simulink model "pendulo"  (R2019b)
settings: Solver=ode45  StartTime=0  StopTime=inf  MaxStep=0.02  RelTol=1e-3  AbsTol=1e-6
libraries: neural x76, simulink x2
(part 2 of 4)

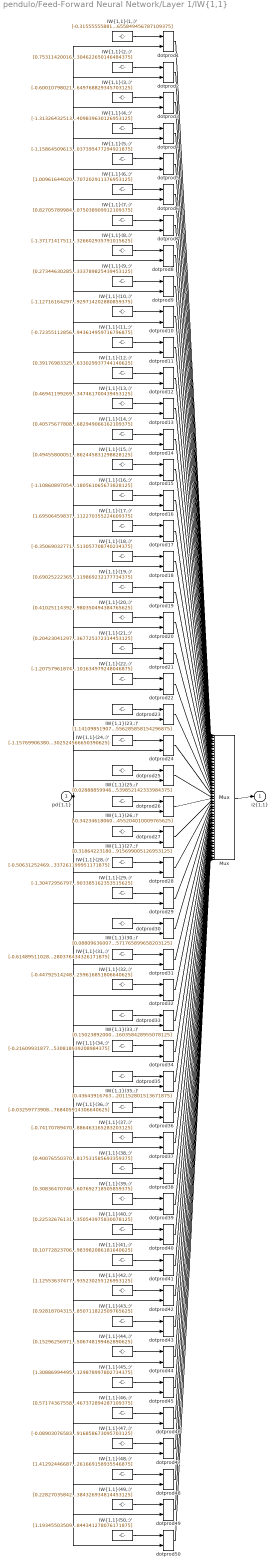
== system pendulo/Feed-Forward Neural Network/Layer 1/IW{1,1} ==
  "pd{1,1}" : Inport  PortDimensions=9
      mask Display: e = 0.06;c1 = [120 230 180]/255;c2 = ([120 230 180]+0)/(256+128);c3 = ([120 230 180]+128)/(256+128);patch([0 1 1 0],[0 0 1 1],c1);patch([0 1 1 1-e 1-e 0+e],[0 0 1 1-e 0+e 0+e],c2);patch([0 0 1 1-e 0+e 0+e],[0 1 1 1-e 1-e 0+e],c3);plot([0 1 1 0 0],[0 0 1 1 0]);
  "IW{1,1}(1,:)'" : Constant  Value=[-0.31555555881384067529182857470004819333553314208984375;0.42878021754571926660304370670928619801998138427734375;-0.0107473012178736886113039616930109332315623760223388671875;-1.3786333332536795381884076050482690334320068359375;0.2466842726358048076829021511002792976796627044677734375;-0.443770337362677957937506789676262997090816497802734375;0.6142590886963574803303345106542110443115234375;0.79347793333041438668118416899233125150203704833984375;0.484092147104690118109004970392561517655849456787109375]
      mask Display: e = 0.06;c1 = [120 150 230]/255;c2 = ([120 150 230]+0)/383;c3 = ([120 150 230]+128)/383;patch([0 1 1 0],[0 0 1 1],c1);patch([0 1 1 1-e 1-e 0+e],[0 0 1 1-e 0+e 0+e],c2);patch([0 0 1 1-e 0+e 0+e],[0 1 1 1-e 1-e 0+e],c3);plot([0 1 1 0 0],[0 0 1 1 0]);disp('Weights');
  "IW{1,1}(10,:)'" : Constant  Value=[-1.127161642979468414438315448933281004428863525390625;-0.01531473256999515801524136549005561391822993755340576171875;0.66738346115575308825640377108356915414333343505859375;0.9754438276149068887121984516852535307407379150390625;-0.9679253878951674661124116028076969087123870849609375;0.733607171987361805776117762434296309947967529296875;0.57226531948503878144407508443691767752170562744140625;-0.931214454864173202253141425899229943752288818359375;0.39431807532208207334178950986824929714202880859375]
      mask Display: e = 0.06;c1 = [120 150 230]/255;c2 = ([120 150 230]+0)/383;c3 = ([120 150 230]+128)/383;patch([0 1 1 0],[0 0 1 1],c1);patch([0 1 1 1-e 1-e 0+e],[0 0 1 1-e 0+e 0+e],c2);patch([0 0 1 1-e 0+e 0+e],[0 1 1 1-e 1-e 0+e],c3);plot([0 1 1 0 0],[0 0 1 1 0]);disp('Weights');
  "IW{1,1}(11,:)'" : Constant  Value=[-0.7235511285626261557268890101113356649875640869140625;-1.1538311728051569016173516502021811902523040771484375;0.83219382713551415253760978885111398994922637939453125;0.8528391957357628339053690069704316556453704833984375;-1.225194887015537137386900212732143700122833251953125;-0.113464709832653609655750415186048485338687896728515625;-0.65765666929837907073164160465239547193050384521484375;-0.6645356436380531750529598866705782711505889892578125;-0.144071189137995492313137901874142698943614959716796875]
      mask Display: e = 0.06;c1 = [120 150 230]/255;c2 = ([120 150 230]+0)/383;c3 = ([120 150 230]+128)/383;patch([0 1 1 0],[0 0 1 1],c1);patch([0 1 1 1-e 1-e 0+e],[0 0 1 1-e 0+e 0+e],c2);patch([0 0 1 1-e 0+e 0+e],[0 1 1 1-e 1-e 0+e],c3);plot([0 1 1 0 0],[0 0 1 1 0]);disp('Weights');
  "IW{1,1}(12,:)'" : Constant  Value=[0.39176983325826231219224382584798149764537811279296875;-0.30969059820905975310978419656748883426189422607421875;-0.157098741820563658766474190997541882097721099853515625;-0.734606532386577359972079648287035524845123291015625;0.2214909422180497688970035596867091953754425048828125;1.28271197347724363879706288571469485759735107421875;0.53025793193026615757190711519797332584857940673828125;0.8886386670511843277608932112343609333038330078125;0.20817546322240121359214981566765345633029937744140625]
      mask Display: e = 0.06;c1 = [120 150 230]/255;c2 = ([120 150 230]+0)/383;c3 = ([120 150 230]+128)/383;patch([0 1 1 0],[0 0 1 1],c1);patch([0 1 1 1-e 1-e 0+e],[0 0 1 1-e 0+e 0+e],c2);patch([0 0 1 1-e 0+e 0+e],[0 1 1 1-e 1-e 0+e],c3);plot([0 1 1 0 0],[0 0 1 1 0]);disp('Weights');
  "IW{1,1}(13,:)'" : Constant  Value=[0.4694119926947788457027854747138917446136474609375;0.84304552135569787996161039700382389128208160400390625;-0.56604187158333540974552988700452260673046112060546875;0.12057132118322488878447984461672604084014892578125;1.928569665412307898577637388370931148529052734375;-0.676114380799501812902008168748579919338226318359375;0.239362492717263009023298536703805439174175262451171875;0.10001219768902032403179447328511741943657398223876953125;-1.3863310520411193937917460061726160347461700439453125]
      mask Display: e = 0.06;c1 = [120 150 230]/255;c2 = ([120 150 230]+0)/383;c3 = ([120 150 230]+128)/383;patch([0 1 1 0],[0 0 1 1],c1);patch([0 1 1 1-e 1-e 0+e],[0 0 1 1-e 0+e 0+e],c2);patch([0 0 1 1-e 0+e 0+e],[0 1 1 1-e 1-e 0+e],c3);plot([0 1 1 0 0],[0 0 1 1 0]);disp('Weights');
  "IW{1,1}(14,:)'" : Constant  Value=[0.405756778086816483064325211671530269086360931396484375;1.4762826494711440705742688805912621319293975830078125;-0.6160052014403716302837210605503059923648834228515625;0.370993442519975957782918385419179685413837432861328125;0.5321273006076394640473381514311768114566802978515625;-0.63250490898227551550547786973766051232814788818359375;0.1763096386724627706588108821961213834583759307861328125;-0.002711608591991353407746334625016970676369965076446533203125;-0.5335206946245099057790639562881551682949066162109375]
      mask Display: e = 0.06;c1 = [120 150 230]/255;c2 = ([120 150 230]+0)/383;c3 = ([120 150 230]+128)/383;patch([0 1 1 0],[0 0 1 1],c1);patch([0 1 1 1-e 1-e 0+e],[0 0 1 1-e 0+e 0+e],c2);patch([0 0 1 1-e 0+e 0+e],[0 1 1 1-e 1-e 0+e],c3);plot([0 1 1 0 0],[0 0 1 1 0]);disp('Weights');
  "IW{1,1}(15,:)'" : Constant  Value=[0.4945580005144349922119317852775566279888153076171875;-0.30371329537800229037003418852691538631916046142578125;-0.12657247648842939735658319477806799113750457763671875;-1.254771661749214839431942891678772866725921630859375;1.2513953241071182898025426766253076493740081787109375;-0.2429382434092005327297414396525709889829158782958984375;-0.9021522058858228998445838442421518266201019287109375;-0.71761308572964221941248297298443503677845001220703125;0.59448766002498942828680128513951785862445831298828125]
      mask Display: e = 0.06;c1 = [120 150 230]/255;c2 = ([120 150 230]+0)/383;c3 = ([120 150 230]+128)/383;patch([0 1 1 0],[0 0 1 1],c1);patch([0 1 1 1-e 1-e 0+e],[0 0 1 1-e 0+e 0+e],c2);patch([0 0 1 1-e 0+e 0+e],[0 1 1 1-e 1-e 0+e],c3);plot([0 1 1 0 0],[0 0 1 1 0]);disp('Weights');
  "IW{1,1}(16,:)'" : Constant  Value=[-1.1086089705421182660671775010996498167514801025390625;0.13153072035216284429992583682178519666194915771484375;0.188915927396714977692937509345938451588153839111328125;-0.8110236400015413682496046021697111427783966064453125;-0.383791213781895346190964346533291973173618316650390625;0.0019837883702850493683467192340685869567096233367919921875;0.68049020551012129320866961279534734785556793212890625;1.2210924520571777573962890528491698205471038818359375;0.9901086444778670614397242388804443180561065673828125]
      mask Display: e = 0.06;c1 = [120 150 230]/255;c2 = ([120 150 230]+0)/383;c3 = ([120 150 230]+128)/383;patch([0 1 1 0],[0 0 1 1],c1);patch([0 1 1 1-e 1-e 0+e],[0 0 1 1-e 0+e 0+e],c2);patch([0 0 1 1-e 0+e 0+e],[0 1 1 1-e 1-e 0+e],c3);plot([0 1 1 0 0],[0 0 1 1 0]);disp('Weights');
  "IW{1,1}(17,:)'" : Constant  Value=[1.695064598379282916340571318869479000568389892578125;0.37882205685793424176921462276368401944637298583984375;0.400870413159026328653311566085903905332088470458984375;-2.0781413995163919850028833025135099887847900390625;1.73490465554027384342816731077618896961212158203125;-1.444554989619908358378097545937635004520416259765625;1.521775698019746325684309340431354939937591552734375;-1.146726490581089219489285824238322675228118896484375;-0.1395995298359869740689731543170637451112270355224609375]
      mask Display: e = 0.06;c1 = [120 150 230]/255;c2 = ([120 150 230]+0)/383;c3 = ([120 150 230]+128)/383;patch([0 1 1 0],[0 0 1 1],c1);patch([0 1 1 1-e 1-e 0+e],[0 0 1 1-e 0+e 0+e],c2);patch([0 0 1 1-e 0+e 0+e],[0 1 1 1-e 1-e 0+e],c3);plot([0 1 1 0 0],[0 0 1 1 0]);disp('Weights');
  "IW{1,1}(18,:)'" : Constant  Value=[-0.350690327718819194746657785799470730125904083251953125;-0.7298307839542406139088370764511637389659881591796875;0.080331001842342708574307152957771904766559600830078125;-0.2264533897417844443555878797269542701542377471923828125;1.2103384853547785038330175666487775743007659912109375;-0.01487761549236282614117055089764107833616435527801513671875;-1.804827730506363803186786753940396010875701904296875;-0.6133682207425008581225256421021185815334320068359375;-1.1075147321910046027682028579874895513057708740234375]
      mask Display: e = 0.06;c1 = [120 150 230]/255;c2 = ([120 150 230]+0)/383;c3 = ([120 150 230]+128)/383;patch([0 1 1 0],[0 0 1 1],c1);patch([0 1 1 1-e 1-e 0+e],[0 0 1 1-e 0+e 0+e],c2);patch([0 0 1 1-e 0+e 0+e],[0 1 1 1-e 1-e 0+e],c3);plot([0 1 1 0 0],[0 0 1 1 0]);disp('Weights');
  "IW{1,1}(19,:)'" : Constant  Value=[0.69025222365466232243846889105043374001979827880859375;0.72407871395070666498128275634371675550937652587890625;-0.9153915604214015733219866888248361647129058837890625;-0.82307459957225870272878864852827973663806915283203125;-0.2295515018585499722458820315296179614961147308349609375;-0.020777463007284745211133980546946986578404903411865234375;-1.7020463564167707115615257862373255193233489990234375;-0.64572237449823177701802023875643499195575714111328125;-0.019957265337930261972498868772163405083119869232177734375]
      mask Display: e = 0.06;c1 = [120 150 230]/255;c2 = ([120 150 230]+0)/383;c3 = ([120 150 230]+128)/383;patch([0 1 1 0],[0 0 1 1],c1);patch([0 1 1 1-e 1-e 0+e],[0 0 1 1-e 0+e 0+e],c2);patch([0 0 1 1-e 0+e 0+e],[0 1 1 1-e 1-e 0+e],c3);plot([0 1 1 0 0],[0 0 1 1 0]);disp('Weights');
  "IW{1,1}(2,:)'" : Constant  Value=[0.75311420016744168304256845658528618514537811279296875;0.79978875953749961613681307426304556429386138916015625;0.96009154060472201575038297960418276488780975341796875;-0.300561830203671165318013436262845061719417572021484375;0.40602009911398384556235896525322459638118743896484375;1.1108934598249404768210979455034248530864715576171875;0.11083407343756877805329708053250215016305446624755859375;1.558741230264542476646738577983342111110687255859375;-0.8332669372419319042677443576394580304622650146484375]
      mask Display: e = 0.06;c1 = [120 150 230]/255;c2 = ([120 150 230]+0)/383;c3 = ([120 150 230]+128)/383;patch([0 1 1 0],[0 0 1 1],c1);patch([0 1 1 1-e 1-e 0+e],[0 0 1 1-e 0+e 0+e],c2);patch([0 0 1 1-e 0+e 0+e],[0 1 1 1-e 1-e 0+e],c3);plot([0 1 1 0 0],[0 0 1 1 0]);disp('Weights');
  "IW{1,1}(20,:)'" : Constant  Value=[0.41025114392726724776849778208998031914234161376953125;-0.94407653012080505749992198616382665932178497314453125;-0.47173289343233426595958235338912345468997955322265625;1.3654696510674215748082360732951201498508453369140625;-0.104760883286913741851975601093727163970470428466796875;1.648557662635401044326499686576426029205322265625;-2.283586288340160752596830207039602100849151611328125;0.78062908761209881536302646054537035524845123291015625;-0.46100003044116155681564350743428803980350494384765625]
      mask Display: e = 0.06;c1 = [120 150 230]/255;c2 = ([120 150 230]+0)/383;c3 = ([120 150 230]+128)/383;patch([0 1 1 0],[0 0 1 1],c1);patch([0 1 1 1-e 1-e 0+e],[0 0 1 1-e 0+e 0+e],c2);patch([0 0 1 1-e 0+e 0+e],[0 1 1 1-e 1-e 0+e],c3);plot([0 1 1 0 0],[0 0 1 1 0]);disp('Weights');
  "IW{1,1}(21,:)'" : Constant  Value=[0.204230412979091335845538424109690822660923004150390625;0.488765287185259966751260662931599654257297515869140625;-0.95418031643023704102546389549388550221920013427734375;0.82964132894869724310638048336841166019439697265625;0.36653691493746032303846504873945377767086029052734375;1.70232992659664006396269542165100574493408203125;-0.37295451432827542159742506555630825459957122802734375;0.383819067928140522649727017778786830604076385498046875;1.0682066467828168487841367095825262367725372314453125]
      mask Display: e = 0.06;c1 = [120 150 230]/255;c2 = ([120 150 230]+0)/383;c3 = ([120 150 230]+128)/383;patch([0 1 1 0],[0 0 1 1],c1);patch([0 1 1 1-e 1-e 0+e],[0 0 1 1-e 0+e 0+e],c2);patch([0 0 1 1-e 0+e 0+e],[0 1 1 1-e 1-e 0+e],c3);plot([0 1 1 0 0],[0 0 1 1 0]);disp('Weights');
  "IW{1,1}(22,:)'" : Constant  Value=[-1.2075796187402361159257679901202209293842315673828125;-1.4344767144320462737283605747506953775882720947265625;-0.385734577372322584576380677390261553227901458740234375;-0.368066024648789624773570494653540663421154022216796875;1.25235491089850103918479362619109451770782470703125;1.395404085665501003887811748427338898181915283203125;0.7191071159702386861312106702825985848903656005859375;0.37835364418729000579588728214730508625507354736328125;-0.55481502754330758175882465366157703101634979248046875]
      mask Display: e = 0.06;c1 = [120 150 230]/255;c2 = ([120 150 230]+0)/383;c3 = ([120 150 230]+128)/383;patch([0 1 1 0],[0 0 1 1],c1);patch([0 1 1 1-e 1-e 0+e],[0 0 1 1-e 0+e 0+e],c2);patch([0 0 1 1-e 0+e 0+e],[0 1 1 1-e 1-e 0+e],c3);plot([0 1 1 0 0],[0 0 1 1 0]);disp('Weights');
  "IW{1,1}(23,:)'" : Constant  Value=[1.141098519073533879009119118563830852508544921875;-0.7222178307753706061333787147304974496364593505859375;-1.0486600899619560323117184452712535858154296875;-0.9834664350422215317593099825899116694927215576171875;0.27914584816355214602623391328961588442325592041015625;-3.002461764557355916593905931222252547740936279296875;0.79946594802184234307418364551267586648464202880859375;-0.291064075115631981649499948616721667349338531494140625;0.266729788638156495306219539997982792556285858154296875]
      mask Display: e = 0.06;c1 = [120 150 230]/255;c2 = ([120 150 230]+0)/383;c3 = ([120 150 230]+128)/383;patch([0 1 1 0],[0 0 1 1],c1);patch([0 1 1 1-e 1-e 0+e],[0 0 1 1-e 0+e 0+e],c2);patch([0 0 1 1-e 0+e 0+e],[0 1 1 1-e 1-e 0+e],c3);plot([0 1 1 0 0],[0 0 1 1 0]);disp('Weights');
  "IW{1,1}(24,:)'" : Constant  Value=[-1.1576990638051898319105248447158373892307281494140625;1.28110704192706226223208432202227413654327392578125;-0.11377994960776420529935393233245122246444225311279296875;0.5335163161567619827252428876818157732486724853515625;-0.5961240722690466231625805448857136070728302001953125;0.1704295245357524135609850191031000576913356781005859375;-2.080284913829131721030307744513265788555145263671875;-0.0464837032769981617352783587193698622286319732666015625;0.11105219603015081819563647513859905302524566650390625]
      mask Display: e = 0.06;c1 = [120 150 230]/255;c2 = ([120 150 230]+0)/383;c3 = ([120 150 230]+128)/383;patch([0 1 1 0],[0 0 1 1],c1);patch([0 1 1 1-e 1-e 0+e],[0 0 1 1-e 0+e 0+e],c2);patch([0 0 1 1-e 0+e 0+e],[0 1 1 1-e 1-e 0+e],c3);plot([0 1 1 0 0],[0 0 1 1 0]);disp('Weights');
  "IW{1,1}(25,:)'" : Constant  Value=[0.0288885994618807394329618176698204479180276393890380859375;0.25905725701129156401947284393827430903911590576171875;0.36959535968647172499146336122066713869571685791015625;-1.06341257201670291721029570908285677433013916015625;-1.1467439713673706069840818599914200603961944580078125;-0.158768234471241276306585632482892833650112152099609375;0.92199159891461934801526467708754353225231170654296875;1.107494697823343532405715450295247137546539306640625;1.587096957328328894476499044685624539852142333984375]
      mask Display: e = 0.06;c1 = [120 150 230]/255;c2 = ([120 150 230]+0)/383;c3 = ([120 150 230]+128)/383;patch([0 1 1 0],[0 0 1 1],c1);patch([0 1 1 1-e 1-e 0+e],[0 0 1 1-e 0+e 0+e],c2);patch([0 0 1 1-e 0+e 0+e],[0 1 1 1-e 1-e 0+e],c3);plot([0 1 1 0 0],[0 0 1 1 0]);disp('Weights');
  "IW{1,1}(26,:)'" : Constant  Value=[-0.342346180602712879537108392469235695898532867431640625;1.5059230527926448228726030720281414687633514404296875;0.832617076855945104085776620195247232913970947265625;-0.470059663377616454571494841729872860014438629150390625;0.64242973391724300658012225540005601942539215087890625;-0.436943685127800407475007204993744380772113800048828125;-1.40624049407380624643337796442210674285888671875;-1.75385756214116472762043486000038683414459228515625;0.120341092838194274605712053016759455204010009765625]
      mask Display: e = 0.06;c1 = [120 150 230]/255;c2 = ([120 150 230]+0)/383;c3 = ([120 150 230]+128)/383;patch([0 1 1 0],[0 0 1 1],c1);patch([0 1 1 1-e 1-e 0+e],[0 0 1 1-e 0+e 0+e],c2);patch([0 0 1 1-e 0+e 0+e],[0 1 1 1-e 1-e 0+e],c3);plot([0 1 1 0 0],[0 0 1 1 0]);disp('Weights');
  "IW{1,1}(27,:)'" : Constant  Value=[0.318642231801257558299056427131290547549724578857421875;-0.675326215282094466374473995529115200042724609375;-0.39831009806688111307693134222063235938549041748046875;0.75477941483355959206846819142811000347137451171875;-0.017647998467868748762032993226966937072575092315673828125;0.44884890348861594677742914427653886377811431884765625;-1.9533747980821474232726586706121452152729034423828125;1.4455729775333920894553330072085373103618621826171875;-0.261998302244357550438991211194661445915699005126953125]
      mask Display: e = 0.06;c1 = [120 150 230]/255;c2 = ([120 150 230]+0)/383;c3 = ([120 150 230]+128)/383;patch([0 1 1 0],[0 0 1 1],c1);patch([0 1 1 1-e 1-e 0+e],[0 0 1 1-e 0+e 0+e],c2);patch([0 0 1 1-e 0+e 0+e],[0 1 1 1-e 1-e 0+e],c3);plot([0 1 1 0 0],[0 0 1 1 0]);disp('Weights');
  "IW{1,1}(28,:)'" : Constant  Value=[-0.506312524694261245628013057284988462924957275390625;-0.90489803148034708701885620030225254595279693603515625;0.71216410228876869670244786902912892401218414306640625;-0.1052561477421264102272147056282847188413143157958984375;0.352357063237664525079395616558031179010868072509765625;-0.378363431434841579470429451248492114245891571044921875;-1.535504428395983556043802309432066977024078369140625;-1.5886664242593286910931738020735792815685272216796875;-0.0152812975359888185422629902632252196781337261199951171875]
      mask Display: e = 0.06;c1 = [120 150 230]/255;c2 = ([120 150 230]+0)/383;c3 = ([120 150 230]+128)/383;patch([0 1 1 0],[0 0 1 1],c1);patch([0 1 1 1-e 1-e 0+e],[0 0 1 1-e 0+e 0+e],c2);patch([0 0 1 1-e 0+e 0+e],[0 1 1 1-e 1-e 0+e],c3);plot([0 1 1 0 0],[0 0 1 1 0]);disp('Weights');
  "IW{1,1}(29,:)'" : Constant  Value=[-1.3047295679785249067350605400861240923404693603515625;0.51214131300232423882334842346608638763427734375;0.9050796768443254425307031851843930780887603759765625;0.61736751265045131109587828177609480917453765869140625;-2.173644167813520322596332334796898066997528076171875;0.65482397329186958767621717925067059695720672607421875;-0.469070913889525653583945086211315356194972991943359375;-0.2988423045945982625681835997966118156909942626953125;0.263423237036322588355830021100700832903385162353515625]
      mask Display: e = 0.06;c1 = [120 150 230]/255;c2 = ([120 150 230]+0)/383;c3 = ([120 150 230]+128)/383;patch([0 1 1 0],[0 0 1 1],c1);patch([0 1 1 1-e 1-e 0+e],[0 0 1 1-e 0+e 0+e],c2);patch([0 0 1 1-e 0+e 0+e],[0 1 1 1-e 1-e 0+e],c3);plot([0 1 1 0 0],[0 0 1 1 0]);disp('Weights');
  "IW{1,1}(3,:)'" : Constant  Value=[-0.60010798021809275137883332718047313392162322998046875;0.918456408957665448866691804141737520694732666015625;-0.488563622390203733392155527326394803822040557861328125;-0.51898886698700408270923389864037744700908660888671875;0.031506951512699055140132031738176010549068450927734375;-0.62720612179891166437784022491541691124439239501953125;-0.167990039071726771080506068756221793591976165771484375;0.66364550463642857369706007375498302280902862548828125;0.44363745867084614094011385532212443649768829345703125]
      mask Display: e = 0.06;c1 = [120 150 230]/255;c2 = ([120 150 230]+0)/383;c3 = ([120 150 230]+128)/383;patch([0 1 1 0],[0 0 1 1],c1);patch([0 1 1 1-e 1-e 0+e],[0 0 1 1-e 0+e 0+e],c2);patch([0 0 1 1-e 0+e 0+e],[0 1 1 1-e 1-e 0+e],c3);plot([0 1 1 0 0],[0 0 1 1 0]);disp('Weights');
  "IW{1,1}(30,:)'" : Constant  Value=[0.088096360074421398156374607424368150532245635986328125;0.125417341018892625204017576834303326904773712158203125;0.80236076444299853083208518000901676714420318603515625;1.4695501105860329094099370195181109011173248291015625;0.493772762787404728701545764124603010714054107666015625;-0.86571053806297670885072648161440156400203704833984375;-0.27053993759736749691313661969616077840328216552734375;0.70993104523678896011773531427024863660335540771484375;0.6738256531354818168466636052471585571765899658203125]
      mask Display: e = 0.06;c1 = [120 150 230]/255;c2 = ([120 150 230]+0)/383;c3 = ([120 150 230]+128)/383;patch([0 1 1 0],[0 0 1 1],c1);patch([0 1 1 1-e 1-e 0+e],[0 0 1 1-e 0+e 0+e],c2);patch([0 0 1 1-e 0+e 0+e],[0 1 1 1-e 1-e 0+e],c3);plot([0 1 1 0 0],[0 0 1 1 0]);disp('Weights');
  "IW{1,1}(31,:)'" : Constant  Value=[-0.61489511028155963145991336205042898654937744140625;-0.454015647212658801645801531776669435203075408935546875;-0.253994370272146607891983194349450059235095977783203125;0.62032010106435520047085674377740360796451568603515625;0.57386932033504389760736330572399310767650604248046875;0.91523673794515281176842336208210326731204986572265625;-2.4057773677357925379283187794499099254608154296875;-0.00117097059544610769543648842727634473703801631927490234375;0.578693589545508757510106079280376434326171875]
      mask Display: e = 0.06;c1 = [120 150 230]/255;c2 = ([120 150 230]+0)/383;c3 = ([120 150 230]+128)/383;patch([0 1 1 0],[0 0 1 1],c1);patch([0 1 1 1-e 1-e 0+e],[0 0 1 1-e 0+e 0+e],c2);patch([0 0 1 1-e 0+e 0+e],[0 1 1 1-e 1-e 0+e],c3);plot([0 1 1 0 0],[0 0 1 1 0]);disp('Weights');
  "IW{1,1}(32,:)'" : Constant  Value=[-0.447925142480680216205968235954060219228267669677734375;1.1636542356515617857581901262165047228336334228515625;0.82724597567363911121418595939758233726024627685546875;-0.548005444646787243101471176487393677234649658203125;-0.63214604842918020732867034894297830760478973388671875;-0.362111865110982755755486550697241909801959991455078125;-0.226400127330656453228385771581088192760944366455078125;-3.298575977733038566697132409899495542049407958984375;-0.2378959620717614742435586094870814122259616851806640625]
      mask Display: e = 0.06;c1 = [120 150 230]/255;c2 = ([120 150 230]+0)/383;c3 = ([120 150 230]+128)/383;patch([0 1 1 0],[0 0 1 1],c1);patch([0 1 1 1-e 1-e 0+e],[0 0 1 1-e 0+e 0+e],c2);patch([0 0 1 1-e 0+e 0+e],[0 1 1 1-e 1-e 0+e],c3);plot([0 1 1 0 0],[0 0 1 1 0]);disp('Weights');
  "IW{1,1}(33,:)'" : Constant  Value=[0.1502389200047310746644058099263929761946201324462890625;0.076394055196631172055532488229800947010517120361328125;0.314550706026246296165282956280861981213092803955078125;1.300730838509452258477949726511724293231964111328125;0.03781352420562822391758572848630137741565704345703125;-0.93135785199220399999120445500011555850505828857421875;1.539524599725752285195312651921994984149932861328125;-0.61418289141405668640771864374983124434947967529296875;-0.282398161560799387803655235984479077160358428955078125]
      mask Display: e = 0.06;c1 = [120 150 230]/255;c2 = ([120 150 230]+0)/383;c3 = ([120 150 230]+128)/383;patch([0 1 1 0],[0 0 1 1],c1);patch([0 1 1 1-e 1-e 0+e],[0 0 1 1-e 0+e 0+e],c2);patch([0 0 1 1-e 0+e 0+e],[0 1 1 1-e 1-e 0+e],c3);plot([0 1 1 0 0],[0 0 1 1 0]);disp('Weights');
  "IW{1,1}(34,:)'" : Constant  Value=[-0.2160993187763598777362261671441956423223018646240234375;-1.016087483009903369435278364107944071292877197265625;0.193857682349798554621855828372645191848278045654296875;0.629272001659570090481565785012207925319671630859375;-0.68828050227516068826361106403055600821971893310546875;2.7608669233230234141274195280857384204864501953125;-1.6160013389992446963816519200918264687061309814453125;2.2825370028224245544379300554282963275909423828125;-0.1709575997603472730101970000760047696530818939208984375]
      mask Display: e = 0.06;c1 = [120 150 230]/255;c2 = ([120 150 230]+0)/383;c3 = ([120 150 230]+128)/383;patch([0 1 1 0],[0 0 1 1],c1);patch([0 1 1 1-e 1-e 0+e],[0 0 1 1-e 0+e 0+e],c2);patch([0 0 1 1-e 0+e 0+e],[0 1 1 1-e 1-e 0+e],c3);plot([0 1 1 0 0],[0 0 1 1 0]);disp('Weights');
  "IW{1,1}(35,:)'" : Constant  Value=[0.436439167633257962819470776594243943691253662109375;-0.066369929598030619199988677792134694755077362060546875;-0.4050231747941259730083629619912244379520416259765625;0.896353825838577034090803863364271819591522216796875;-0.5539314361456373347891712910495698451995849609375;1.347896124115690152933666468015871942043304443359375;-0.102425058063205731695433087224955670535564422607421875;-0.65807979313985554004062805688590742647647857666015625;-0.93098274718173967823275916089187376201152801513671875]
      mask Display: e = 0.06;c1 = [120 150 230]/255;c2 = ([120 150 230]+0)/383;c3 = ([120 150 230]+128)/383;patch([0 1 1 0],[0 0 1 1],c1);patch([0 1 1 1-e 1-e 0+e],[0 0 1 1-e 0+e 0+e],c2);patch([0 0 1 1-e 0+e 0+e],[0 1 1 1-e 1-e 0+e],c3);plot([0 1 1 0 0],[0 0 1 1 0]);disp('Weights');
  "IW{1,1}(36,:)'" : Constant  Value=[-0.032597739080619310414466127667765249498188495635986328125;0.00940020588488926951697965961329828132875263690948486328125;-1.5630841184982318115004318315186537802219390869140625;-1.0623572721555671893867156541091389954090118408203125;1.5897937578240759481928989771404303610324859619140625;1.6593572786997270451792019230197183787822723388671875;-1.0581794050147530494854208882316015660762786865234375;-0.5993642744934184474203675563330762088298797607421875;-0.120486966060517064480706039830693043768405914306640625]
      mask Display: e = 0.06;c1 = [120 150 230]/255;c2 = ([120 150 230]+0)/383;c3 = ([120 150 230]+128)/383;patch([0 1 1 0],[0 0 1 1],c1);patch([0 1 1 1-e 1-e 0+e],[0 0 1 1-e 0+e 0+e],c2);patch([0 0 1 1-e 0+e 0+e],[0 1 1 1-e 1-e 0+e],c3);plot([0 1 1 0 0],[0 0 1 1 0]);disp('Weights');
  "IW{1,1}(37,:)'" : Constant  Value=[-0.7417078947075037564928834399324841797351837158203125;-1.4642032757034570966681030768086202442646026611328125;-0.441811921591786338492369168307050131261348724365234375;0.6677734635750933733788770041428506374359130859375;-0.8910019354307074923582376868580467998981475830078125;-0.95395879175244957526302869155188091099262237548828125;-2.664186918615282895217433178913779556751251220703125;1.2975226196660887278966356461751274764537811279296875;0.265215194162956191537006134240073151886463165283203125]
      mask Display: e = 0.06;c1 = [120 150 230]/255;c2 = ([120 150 230]+0)/383;c3 = ([120 150 230]+128)/383;patch([0 1 1 0],[0 0 1 1],c1);patch([0 1 1 1-e 1-e 0+e],[0 0 1 1-e 0+e 0+e],c2);patch([0 0 1 1-e 0+e 0+e],[0 1 1 1-e 1-e 0+e],c3);plot([0 1 1 0 0],[0 0 1 1 0]);disp('Weights');
  "IW{1,1}(38,:)'" : Constant  Value=[0.400765503705490189201299244814435951411724090576171875;0.50526638806091328515179839087068103253841400146484375;-1.2536405658766500703649171555298380553722381591796875;-1.07783516630355524767992392298765480518341064453125;0.65331900037182466522978074863203801214694976806640625;0.16422468634164866241320623885258100926876068115234375;1.0099526480469120937044635866186581552028656005859375;0.7291633231945269244533847086131572723388671875;-0.4454084174562209508252408340922556817531585693359375]
      mask Display: e = 0.06;c1 = [120 150 230]/255;c2 = ([120 150 230]+0)/383;c3 = ([120 150 230]+128)/383;patch([0 1 1 0],[0 0 1 1],c1);patch([0 1 1 1-e 1-e 0+e],[0 0 1 1-e 0+e 0+e],c2);patch([0 0 1 1-e 0+e 0+e],[0 1 1 1-e 1-e 0+e],c3);plot([0 1 1 0 0],[0 0 1 1 0]);disp('Weights');
  "IW{1,1}(39,:)'" : Constant  Value=[0.30836470746044086777004622490494512021541595458984375;-0.9461172142420519737271433768910355865955352783203125;-0.61612646247528568554940875401371158659458160400390625;0.31716226887904586106969873071648180484771728515625;-0.189342552119727558501693920334219001233577728271484375;1.7621747274356227563885113340802490711212158203125;-1.7636440394071775106255017817602492868900299072265625;0.53617770408947673654864729542168788611888885498046875;0.6834329148339788329025168422958813607692718505859375]
      mask Display: e = 0.06;c1 = [120 150 230]/255;c2 = ([120 150 230]+0)/383;c3 = ([120 150 230]+128)/383;patch([0 1 1 0],[0 0 1 1],c1);patch([0 1 1 1-e 1-e 0+e],[0 0 1 1-e 0+e 0+e],c2);patch([0 0 1 1-e 0+e 0+e],[0 1 1 1-e 1-e 0+e],c3);plot([0 1 1 0 0],[0 0 1 1 0]);disp('Weights');
  "IW{1,1}(4,:)'" : Constant  Value=[-1.313264325139350763294032731209881603717803955078125;0.577430178245246228385667563998140394687652587890625;0.59261872570352291944573153159581124782562255859375;1.1565928017486708512251425418071448802947998046875;-1.5158360318740642380674898959114216268062591552734375;0.23944884577022051974637406601686961948871612548828125;-0.741730729462697357945444309734739363193511962890625;-0.49748483589540148930296936669037677347660064697265625;-1.0698272503985439829676806766656227409839630126953125]
      mask Display: e = 0.06;c1 = [120 150 230]/255;c2 = ([120 150 230]+0)/383;c3 = ([120 150 230]+128)/383;patch([0 1 1 0],[0 0 1 1],c1);patch([0 1 1 1-e 1-e 0+e],[0 0 1 1-e 0+e 0+e],c2);patch([0 0 1 1-e 0+e 0+e],[0 1 1 1-e 1-e 0+e],c3);plot([0 1 1 0 0],[0 0 1 1 0]);disp('Weights');
  "IW{1,1}(40,:)'" : Constant  Value=[0.2253267613164235683154146272499929182231426239013671875;-0.72744873942601151473041909412131644785404205322265625;0.494167563515222230119405821824329905211925506591796875;1.1645096904818676986081982249743305146694183349609375;1.354357965548462328086998240905813872814178466796875;0.515846662339619843606897120480425655841827392578125;-2.991249228996013531656217310228385031223297119140625;-0.5807989748192843304508414803422056138515472412109375;-0.84618756083541335488718004853581078350543975830078125]
      mask Display: e = 0.06;c1 = [120 150 230]/255;c2 = ([120 150 230]+0)/383;c3 = ([120 150 230]+128)/383;patch([0 1 1 0],[0 0 1 1],c1);patch([0 1 1 1-e 1-e 0+e],[0 0 1 1-e 0+e 0+e],c2);patch([0 0 1 1-e 0+e 0+e],[0 1 1 1-e 1-e 0+e],c3);plot([0 1 1 0 0],[0 0 1 1 0]);disp('Weights');
  "IW{1,1}(41,:)'" : Constant  Value=[0.107728237063276555129931466581183485686779022216796875;-0.404281704316281242927999528546934016048908233642578125;1.4955745902677739511688059792504645884037017822265625;0.060690974968412504664261319931028992868959903717041015625;0.287713764701010232816003053812892176210880279541015625;0.7331962147546924324359451929922215640544891357421875;0.86318088328563080668942575357505120337009429931640625;1.5812769879263697259119680893491022288799285888671875;-0.36577143068486750454582079328247345983982086181640625]
      mask Display: e = 0.06;c1 = [120 150 230]/255;c2 = ([120 150 230]+0)/383;c3 = ([120 150 230]+128)/383;patch([0 1 1 0],[0 0 1 1],c1);patch([0 1 1 1-e 1-e 0+e],[0 0 1 1-e 0+e 0+e],c2);patch([0 0 1 1-e 0+e 0+e],[0 1 1 1-e 1-e 0+e],c3);plot([0 1 1 0 0],[0 0 1 1 0]);disp('Weights');
  "IW{1,1}(42,:)'" : Constant  Value=[1.1255363747790969597417642944492399692535400390625;-0.025706183688733001690973622999081271700561046600341796875;-0.484981238223346100557620275139925070106983184814453125;-0.98625569121625122903651572414673864841461181640625;0.03753959977101918588093809603378758765757083892822265625;-1.00586934735876720736769129871390759944915771484375;0.5739751137437598682566886054701171815395355224609375;0.775221131153772002875257385312579572200775146484375;-0.61105789315256064941905833620694465935230255126953125]
      mask Display: e = 0.06;c1 = [120 150 230]/255;c2 = ([120 150 230]+0)/383;c3 = ([120 150 230]+128)/383;patch([0 1 1 0],[0 0 1 1],c1);patch([0 1 1 1-e 1-e 0+e],[0 0 1 1-e 0+e 0+e],c2);patch([0 0 1 1-e 0+e 0+e],[0 1 1 1-e 1-e 0+e],c3);plot([0 1 1 0 0],[0 0 1 1 0]);disp('Weights');
  "IW{1,1}(43,:)'" : Constant  Value=[0.92818704315667588389260345138609409332275390625;0.00866950617375148065157919319290158455260097980499267578125;-0.64008262890003908562874812560039572417736053466796875;-0.8548217496565875261893552305991761386394500732421875;-0.2402185911989817290734805510510341264307498931884765625;-1.495915794684951283244345177081413567066192626953125;1.8430815049572377706255110751953907310962677001953125;-1.5968541049881306292945737368427217006683349609375;-0.91335899636081185892777511980966664850711822509765625]
      mask Display: e = 0.06;c1 = [120 150 230]/255;c2 = ([120 150 230]+0)/383;c3 = ([120 150 230]+128)/383;patch([0 1 1 0],[0 0 1 1],c1);patch([0 1 1 1-e 1-e 0+e],[0 0 1 1-e 0+e 0+e],c2);patch([0 0 1 1-e 0+e 0+e],[0 1 1 1-e 1-e 0+e],c3);plot([0 1 1 0 0],[0 0 1 1 0]);disp('Weights');
  "IW{1,1}(44,:)'" : Constant  Value=[0.1529625697167308062685009417691617272794246673583984375;0.97732281546550925366290130114066414535045623779296875;-0.56278454962883817103147521265782415866851806640625;-0.52553410103238740180842114568804390728473663330078125;-0.85806568612284817021418348303996026515960693359375;0.7445806319677148454871939975419081747531890869140625;-0.256530000406411329283429267889005132019519805908203125;0.8075865545580906967870760126970708370208740234375;-0.4874945042220029112201018506311811506748199462890625]
      mask Display: e = 0.06;c1 = [120 150 230]/255;c2 = ([120 150 230]+0)/383;c3 = ([120 150 230]+128)/383;patch([0 1 1 0],[0 0 1 1],c1);patch([0 1 1 1-e 1-e 0+e],[0 0 1 1-e 0+e 0+e],c2);patch([0 0 1 1-e 0+e 0+e],[0 1 1 1-e 1-e 0+e],c3);plot([0 1 1 0 0],[0 0 1 1 0]);disp('Weights');
  "IW{1,1}(45,:)'" : Constant  Value=[1.3088699449507092964495313935913145542144775390625;0.64354427196952179723865583582664839923381805419921875;-0.6964658495650899450168935800320468842983245849609375;-0.208199507696994190464323537526070140302181243896484375;0.846978807405621036963339065550826489925384521484375;0.5947279136631979934435321411001496016979217529296875;1.0204117795934217749476147218956612050533294677734375;0.060045353954537368512678341403443482704460620880126953125;-0.57534331505092006775470281354500912129878997802734375]
      mask Display: e = 0.06;c1 = [120 150 230]/255;c2 = ([120 150 230]+0)/383;c3 = ([120 150 230]+128)/383;patch([0 1 1 0],[0 0 1 1],c1);patch([0 1 1 1-e 1-e 0+e],[0 0 1 1-e 0+e 0+e],c2);patch([0 0 1 1-e 0+e 0+e],[0 1 1 1-e 1-e 0+e],c3);plot([0 1 1 0 0],[0 0 1 1 0]);disp('Weights');
  "IW{1,1}(46,:)'" : Constant  Value=[0.57174367558978411718584311529411934316158294677734375;-0.464679428478108003108815182713442482054233551025390625;-0.6170736426773031357839727206737734377384185791015625;-1.63257715473088627078368517686612904071807861328125;0.46912969929478653963172973817563615739345550537109375;-0.328500661122216708331933432418736629188060760498046875;-0.57585633025811555629758231589221395552158355712890625;0.1860662669392543211444035478052683174610137939453125;-0.52011575757743278014544330289936624467372894287109375]
      mask Display: e = 0.06;c1 = [120 150 230]/255;c2 = ([120 150 230]+0)/383;c3 = ([120 150 230]+128)/383;patch([0 1 1 0],[0 0 1 1],c1);patch([0 1 1 1-e 1-e 0+e],[0 0 1 1-e 0+e 0+e],c2);patch([0 0 1 1-e 0+e 0+e],[0 1 1 1-e 1-e 0+e],c3);plot([0 1 1 0 0],[0 0 1 1 0]);disp('Weights');
  "IW{1,1}(47,:)'" : Constant  Value=[-0.089030765831632552309571337900706566870212554931640625;-0.75483625801540521482735357494675554335117340087890625;0.0394836553850045623992315313444123603403568267822265625;0.64829089224797253887544457029434852302074432373046875;-0.27305487478529599787435699909110553562641143798828125;-0.9162924501737725879735307898954488337039947509765625;-1.239579832779849954960127433878369629383087158203125;1.6201087438132451001848721716669388115406036376953125;0.93580501954427230959510097818565554916858673095703125]
      mask Display: e = 0.06;c1 = [120 150 230]/255;c2 = ([120 150 230]+0)/383;c3 = ([120 150 230]+128)/383;patch([0 1 1 0],[0 0 1 1],c1);patch([0 1 1 1-e 1-e 0+e],[0 0 1 1-e 0+e 0+e],c2);patch([0 0 1 1-e 0+e 0+e],[0 1 1 1-e 1-e 0+e],c3);plot([0 1 1 0 0],[0 0 1 1 0]);disp('Weights');
  "IW{1,1}(48,:)'" : Constant  Value=[1.4129244668716400834540536379790864884853363037109375;0.1354011458253276678487253548155422322452068328857421875;-0.51830764909016446839729042039834894239902496337890625;0.72432435951206175506200679592438973486423492431640625;-0.463203984082069364358602570064249448478221893310546875;-1.420163917436811029659793348400853574275970458984375;1.78534580440193213490829293732531368732452392578125;-0.493841080149864442017104693150031380355358123779296875;0.0453350343107105924200794788703205995261669158935546875]
      mask Display: e = 0.06;c1 = [120 150 230]/255;c2 = ([120 150 230]+0)/383;c3 = ([120 150 230]+128)/383;patch([0 1 1 0],[0 0 1 1],c1);patch([0 1 1 1-e 1-e 0+e],[0 0 1 1-e 0+e 0+e],c2);patch([0 0 1 1-e 0+e 0+e],[0 1 1 1-e 1-e 0+e],c3);plot([0 1 1 0 0],[0 0 1 1 0]);disp('Weights');
  "IW{1,1}(49,:)'" : Constant  Value=[0.2282703584214630099236131854922859929502010345458984375;-0.3153756464550985239014835315174423158168792724609375;-0.0967401052640957381800745906730298884212970733642578125;-0.1848623589101048569904861551549402065575122833251953125;-0.348643515079936516798397860839031636714935302734375;-1.2152883840003647630823024883284233510494232177734375;-0.2131748800712598701512234811161761172115802764892578125;1.2849396870758791333599901918205432593822479248046875;0.428082449189977343184665414810297079384326934814453125]
      mask Display: e = 0.06;c1 = [120 150 230]/255;c2 = ([120 150 230]+0)/383;c3 = ([120 150 230]+128)/383;patch([0 1 1 0],[0 0 1 1],c1);patch([0 1 1 1-e 1-e 0+e],[0 0 1 1-e 0+e 0+e],c2);patch([0 0 1 1-e 0+e 0+e],[0 1 1 1-e 1-e 0+e],c3);plot([0 1 1 0 0],[0 0 1 1 0]);disp('Weights');
  "IW{1,1}(5,:)'" : Constant  Value=[-1.1586450961340972742874555478920228779315948486328125;0.86603543464462429124495201904210262000560760498046875;-0.98898542847015102896790494924061931669712066650390625;-0.71856379014599747190317202694131992757320404052734375;-0.957587367793592658671286699245683848857879638671875;-0.27196898103878097696650684156338684260845184326171875;0.54967310437313143811621785062015987932682037353515625;0.456219509012878055020934198182658292353153228759765625;0.61646496004982231919910873330081813037395477294921875]
      mask Display: e = 0.06;c1 = [120 150 230]/255;c2 = ([120 150 230]+0)/383;c3 = ([120 150 230]+128)/383;patch([0 1 1 0],[0 0 1 1],c1);patch([0 1 1 1-e 1-e 0+e],[0 0 1 1-e 0+e 0+e],c2);patch([0 0 1 1-e 0+e 0+e],[0 1 1 1-e 1-e 0+e],c3);plot([0 1 1 0 0],[0 0 1 1 0]);disp('Weights');
  "IW{1,1}(50,:)'" : Constant  Value=[1.193455035090516869189514181925915181636810302734375;-0.07137178442131568434358968033848213963210582733154296875;-0.343478174381469492093543749433592893183231353759765625;-0.6739219251907597740824940046877600252628326416015625;0.32778546147606657523709827728453092277050018310546875;-1.07881066144221282598891775705851614475250244140625;0.91057454245496283196104059243225492537021636962890625;-1.56155142279065817234595670015551149845123291015625;-1.6620785833296352063115364217082969844341278076171875]
      mask Display: e = 0.06;c1 = [120 150 230]/255;c2 = ([120 150 230]+0)/383;c3 = ([120 150 230]+128)/383;patch([0 1 1 0],[0 0 1 1],c1);patch([0 1 1 1-e 1-e 0+e],[0 0 1 1-e 0+e 0+e],c2);patch([0 0 1 1-e 0+e 0+e],[0 1 1 1-e 1-e 0+e],c3);plot([0 1 1 0 0],[0 0 1 1 0]);disp('Weights');
  "IW{1,1}(6,:)'" : Constant  Value=[1.0096164402001150950383134841104038059711456298828125;-0.5087921797833383497078330037766136229038238525390625;-0.282530570280445536557323293891386128962039947509765625;0.72584013128025526295772351659252308309078216552734375;-1.6716593354462292442264015335240401327610015869140625;0.372859509415361001227751103215268813073635101318359375;-1.11998938506951351001816874486394226551055908203125;-0.97809014605269961606381912133656442165374755859375;-0.5565014473732905475600318823126144707202911376953125]
      mask Display: e = 0.06;c1 = [120 150 230]/255;c2 = ([120 150 230]+0)/383;c3 = ([120 150 230]+128)/383;patch([0 1 1 0],[0 0 1 1],c1);patch([0 1 1 1-e 1-e 0+e],[0 0 1 1-e 0+e 0+e],c2);patch([0 0 1 1-e 0+e 0+e],[0 1 1 1-e 1-e 0+e],c3);plot([0 1 1 0 0],[0 0 1 1 0]);disp('Weights');
  "IW{1,1}(7,:)'" : Constant  Value=[0.82705789984217659149834389609168283641338348388671875;-0.91517933332349510333614261980983428657054901123046875;-1.1887679105232697995830903892056085169315338134765625;0.325102448305115976356916007716790772974491119384765625;-1.694022640331411810876716117491014301776885986328125;-1.7891524794039970203129996662028133869171142578125;1.4183468714626688012003796757198870182037353515625;-0.428883561134236479528425434182281605899333953857421875;-0.1994797803117468182332316928295767866075038909912109375]
      mask Display: e = 0.06;c1 = [120 150 230]/255;c2 = ([120 150 230]+0)/383;c3 = ([120 150 230]+128)/383;patch([0 1 1 0],[0 0 1 1],c1);patch([0 1 1 1-e 1-e 0+e],[0 0 1 1-e 0+e 0+e],c2);patch([0 0 1 1-e 0+e 0+e],[0 1 1 1-e 1-e 0+e],c3);plot([0 1 1 0 0],[0 0 1 1 0]);disp('Weights');
  "IW{1,1}(8,:)'" : Constant  Value=[-1.3717141751145340844431075311149470508098602294921875;-0.16600636872701624024983857452752999961376190185546875;-0.0175566148612653870342281692273900262080132961273193359375;-0.39982736491193182626346924735116772353649139404296875;-0.3126907004793497701911064723390154540538787841796875;0.90728952553643704703745243023149669170379638671875;-0.93880271077071519858492365528945811092853546142578125;0.77296319069262953149745953851379454135894775390625;-0.9773491125384110578266927404911257326602935791015625]
      mask Display: e = 0.06;c1 = [120 150 230]/255;c2 = ([120 150 230]+0)/383;c3 = ([120 150 230]+128)/383;patch([0 1 1 0],[0 0 1 1],c1);patch([0 1 1 1-e 1-e 0+e],[0 0 1 1-e 0+e 0+e],c2);patch([0 0 1 1-e 0+e 0+e],[0 1 1 1-e 1-e 0+e],c3);plot([0 1 1 0 0],[0 0 1 1 0]);disp('Weights');
  "IW{1,1}(9,:)'" : Constant  Value=[0.2734463028534468431729465009993873536586761474609375;-0.80819905082407961227630721623427234590053558349609375;-0.42058233299171454699916239405865781009197235107421875;0.10067193516282983700715902841693605296313762664794921875;0.376730661079810180691396226393408142030239105224609375;0.76916785552568944783757842742488719522953033447265625;1.4174229167593725975393681437708437442779541015625;-1.448093410453322515962781835696659982204437255859375;0.335864564909991447638759609617409296333789825439453125]
      mask Display: e = 0.06;c1 = [120 150 230]/255;c2 = ([120 150 230]+0)/383;c3 = ([120 150 230]+128)/383;patch([0 1 1 0],[0 0 1 1],c1);patch([0 1 1 1-e 1-e 0+e],[0 0 1 1-e 0+e 0+e],c2);patch([0 0 1 1-e 0+e 0+e],[0 1 1 1-e 1-e 0+e],c3);plot([0 1 1 0 0],[0 0 1 1 0]);disp('Weights');
  Mux : Mux  Inputs=50
      mask Display: e = 0.06;c1 = [120 150 230]/255;c2 = ([120 150 230]+0)/383;c3 = ([120 150 230]+128)/383;patch([0 1 1 0],[0 0 1 1],c1);patch([0 1 1 1-e 1-e 0+e],[0 0 1 1-e 0+e 0+e],c2);patch([0 0 1 1-e 0+e 0+e],[0 1 1 1-e 1-e 0+e],c3);plot([0 1 1 0 0],[0 0 1 1 0]);disp('Mux');
  dotprod{1..50} (50 alike) : neural/Weight Functions/dotprod
      settings: SourceProductName=Deep Learning Toolbox
  "iz{1,1}" : Outport
      mask Display: e = 0.06;c1 = [120 230 180]/255;c2 = ([120 230 180]+0)/(256+128);c3 = ([120 230 180]+128)/(256+128);patch([0 1 1 0],[0 0 1 1],c1);patch([0 1 1 1-e 1-e 0+e],[0 0 1 1-e 0+e 0+e],c2);patch([0 0 1 1-e 0+e 0+e],[0 1 1 1-e 1-e 0+e],c3);plot([0 1 1 0 0],[0 0 1 1 0]);
  wires:
  "IW{1,1}(1,:)'"/1 -> dotprod1/1
  "pd{1,1}"/1 -> dotprod1/2, dotprod2/2, dotprod3/2, dotprod4/2, dotprod5/2, dotprod6/2, dotprod7/2, dotprod8/2, dotprod9/2, dotprod10/2, dotprod11/2, dotprod12/2, dotprod13/2, dotprod14/2, dotprod15/2, dotprod16/2, dotprod17/2, dotprod18/2, dotprod19/2, dotprod20/2, dotprod21/2, dotprod22/2, dotprod23/2, dotprod24/2, dotprod25/2, dotprod26/2, dotprod27/2, dotprod28/2, dotprod29/2, dotprod30/2, dotprod31/2, dotprod32/2, dotprod33/2, dotprod34/2, dotprod35/2, dotprod36/2, dotprod37/2, dotprod38/2, dotprod39/2, dotprod40/2, dotprod41/2, dotprod42/2, dotprod43/2, dotprod44/2, dotprod45/2, dotprod46/2, dotprod47/2, dotprod48/2, dotprod49/2, dotprod50/2
  dotprod1/1 -> Mux/1
  "IW{1,1}(2,:)'"/1 -> dotprod2/1
  dotprod2/1 -> Mux/2
  "IW{1,1}(3,:)'"/1 -> dotprod3/1
  dotprod3/1 -> Mux/3
  "IW{1,1}(4,:)'"/1 -> dotprod4/1
  dotprod4/1 -> Mux/4
  "IW{1,1}(5,:)'"/1 -> dotprod5/1
  dotprod5/1 -> Mux/5
  "IW{1,1}(6,:)'"/1 -> dotprod6/1
  dotprod6/1 -> Mux/6
  "IW{1,1}(7,:)'"/1 -> dotprod7/1
  dotprod7/1 -> Mux/7
  "IW{1,1}(8,:)'"/1 -> dotprod8/1
  dotprod8/1 -> Mux/8
  "IW{1,1}(9,:)'"/1 -> dotprod9/1
  dotprod9/1 -> Mux/9
  "IW{1,1}(10,:)'"/1 -> dotprod10/1
  dotprod10/1 -> Mux/10
  "IW{1,1}(11,:)'"/1 -> dotprod11/1
  dotprod11/1 -> Mux/11
  "IW{1,1}(12,:)'"/1 -> dotprod12/1
  dotprod12/1 -> Mux/12
  "IW{1,1}(13,:)'"/1 -> dotprod13/1
  dotprod13/1 -> Mux/13
  "IW{1,1}(14,:)'"/1 -> dotprod14/1
  dotprod14/1 -> Mux/14
  "IW{1,1}(15,:)'"/1 -> dotprod15/1
  dotprod15/1 -> Mux/15
  "IW{1,1}(16,:)'"/1 -> dotprod16/1
  dotprod16/1 -> Mux/16
  "IW{1,1}(17,:)'"/1 -> dotprod17/1
  dotprod17/1 -> Mux/17
  "IW{1,1}(18,:)'"/1 -> dotprod18/1
  dotprod18/1 -> Mux/18
  "IW{1,1}(19,:)'"/1 -> dotprod19/1
  dotprod19/1 -> Mux/19
  "IW{1,1}(20,:)'"/1 -> dotprod20/1
  dotprod20/1 -> Mux/20
  "IW{1,1}(21,:)'"/1 -> dotprod21/1
  dotprod21/1 -> Mux/21
  "IW{1,1}(22,:)'"/1 -> dotprod22/1
  dotprod22/1 -> Mux/22
  "IW{1,1}(23,:)'"/1 -> dotprod23/1
  dotprod23/1 -> Mux/23
  "IW{1,1}(24,:)'"/1 -> dotprod24/1
  dotprod24/1 -> Mux/24
  "IW{1,1}(25,:)'"/1 -> dotprod25/1
  dotprod25/1 -> Mux/25
  "IW{1,1}(26,:)'"/1 -> dotprod26/1
  dotprod26/1 -> Mux/26
  "IW{1,1}(27,:)'"/1 -> dotprod27/1
  dotprod27/1 -> Mux/27
  "IW{1,1}(28,:)'"/1 -> dotprod28/1
  dotprod28/1 -> Mux/28
  "IW{1,1}(29,:)'"/1 -> dotprod29/1
  dotprod29/1 -> Mux/29
  "IW{1,1}(30,:)'"/1 -> dotprod30/1
  dotprod30/1 -> Mux/30
  "IW{1,1}(31,:)'"/1 -> dotprod31/1
  dotprod31/1 -> Mux/31
  "IW{1,1}(32,:)'"/1 -> dotprod32/1
  dotprod32/1 -> Mux/32
  "IW{1,1}(33,:)'"/1 -> dotprod33/1
  dotprod33/1 -> Mux/33
  "IW{1,1}(34,:)'"/1 -> dotprod34/1
  dotprod34/1 -> Mux/34
  "IW{1,1}(35,:)'"/1 -> dotprod35/1
  dotprod35/1 -> Mux/35
  "IW{1,1}(36,:)'"/1 -> dotprod36/1
  dotprod36/1 -> Mux/36
  "IW{1,1}(37,:)'"/1 -> dotprod37/1
  dotprod37/1 -> Mux/37
  "IW{1,1}(38,:)'"/1 -> dotprod38/1
  dotprod38/1 -> Mux/38
  "IW{1,1}(39,:)'"/1 -> dotprod39/1
  dotprod39/1 -> Mux/39
  "IW{1,1}(40,:)'"/1 -> dotprod40/1
  dotprod40/1 -> Mux/40
  "IW{1,1}(41,:)'"/1 -> dotprod41/1
  dotprod41/1 -> Mux/41
  "IW{1,1}(42,:)'"/1 -> dotprod42/1
  dotprod42/1 -> Mux/42
  "IW{1,1}(43,:)'"/1 -> dotprod43/1
  dotprod43/1 -> Mux/43
  "IW{1,1}(44,:)'"/1 -> dotprod44/1
  dotprod44/1 -> Mux/44
  "IW{1,1}(45,:)'"/1 -> dotprod45/1
  dotprod45/1 -> Mux/45
  "IW{1,1}(46,:)'"/1 -> dotprod46/1
  dotprod46/1 -> Mux/46
  "IW{1,1}(47,:)'"/1 -> dotprod47/1
  dotprod47/1 -> Mux/47
  "IW{1,1}(48,:)'"/1 -> dotprod48/1
  dotprod48/1 -> Mux/48
  "IW{1,1}(49,:)'"/1 -> dotprod49/1
  dotprod49/1 -> Mux/49
  "IW{1,1}(50,:)'"/1 -> dotprod50/1
  dotprod50/1 -> Mux/50
  Mux/1 -> "iz{1,1}"/1

== system pendulo/Feed-Forward Neural Network/Layer 2/Delays 1 ==
  "p{2}" : Inport  PortDimensions=50
      mask Display: e = 0.06;c1 = [120 230 180]/255;c2 = ([120 230 180]+0)/(256+128);c3 = ([120 230 180]+128)/(256+128);patch([0 1 1 0],[0 0 1 1],c1);patch([0 1 1 1-e 1-e 0+e],[0 0 1 1-e 0+e 0+e],c2);patch([0 0 1 1-e 0+e 0+e],[0 1 1 1-e 1-e 0+e],c3);plot([0 1 1 0 0],[0 0 1 1 0]);
  mux : Mux  Inputs=1
      mask Display: e = 0.06;c1 = [120 150 230]/255;c2 = ([120 150 230]+0)/383;c3 = ([120 150 230]+128)/383;patch([0 1 1 0],[0 0 1 1],c1);patch([0 1 1 1-e 1-e 0+e],[0 0 1 1-e 0+e 0+e],c2);patch([0 0 1 1-e 0+e 0+e],[0 1 1 1-e 1-e 0+e],c3);plot([0 1 1 0 0],[0 0 1 1 0]);disp('Mux')
  "pd{2,1}" : Outport
      mask Display: e = 0.06;c1 = [120 230 180]/255;c2 = ([120 230 180]+0)/(256+128);c3 = ([120 230 180]+128)/(256+128);patch([0 1 1 0],[0 0 1 1],c1);patch([0 1 1 1-e 1-e 0+e],[0 0 1 1-e 0+e 0+e],c2);patch([0 0 1 1-e 0+e 0+e],[0 1 1 1-e 1-e 0+e],c3);plot([0 1 1 0 0],[0 0 1 1 0]);
  wires:
  "p{2}"/1 -> mux/1
  mux/1 -> "pd{2,1}"/1
